simulink model "Newtons"  (R2020b)
settings: Solver=VariableStepAuto  StartTime=0.0  StopTime=60  RelTol=1e-3
settings Model: Creator=jimd  LastModifiedBy=jimd

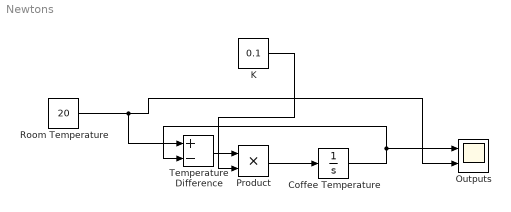
== system Newtons ==
  Coffee Temperature : Integrator  InitialCondition=4
  K : Constant  Value=0.1
  Outputs : Scope  NumInputPorts=2
  Product : Product
  Room Temperature : Constant  Value=20
  Temperature Difference : Sum  Inputs=+-
  wires:
  K/1 -> Product/2
  Product/1 -> Coffee Temperature/1
  Temperature Difference/1 -> Product/1
  Coffee Temperature/1 -> Temperature Difference/2, Outputs/1
  Room Temperature/1 -> Temperature Difference/1, Outputs/2
